simulink model "Harness_chart2"  (R2017b)
settings: Solver=VariableStepAuto  StartTime=0.0  StopTime=2  RelTol=1e-3
undefined symbols (not defined in the file): sigbuilder_block
settings Model: Creator=Kris  LastModifiedBy=Kris

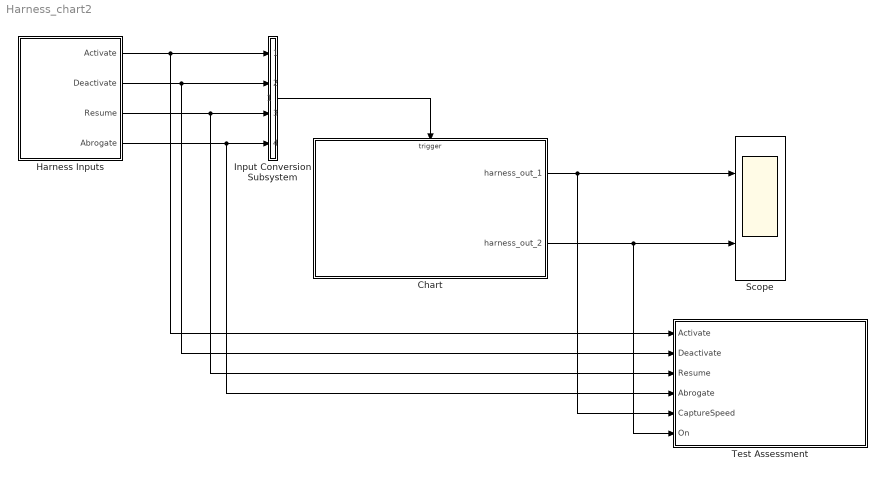
== system Harness_chart2 ==
  Chart : Subsystem  Tag=__SL_testing_harness_stub_
  Harness Inputs : Subsystem  Tag=STV Subsys  LoadFcn=sigbuilder_block('load');  StartFcn=sigbuilder_block('start');  StopFcn=sigbuilder_block('stop');  ClipboardFcn=sigbuilder_block('clipboard');  mask(Sigbuilder block){tuvar=[0:10]}
      mask init:
      | if ~strcmp(get_param(bdroot(gcb),'SimulationStatus'),'stopped'),tuvar = sigbuilder_block('maskInit'); end
      settings: CopyFcn=sigbuilder_block('copy');  DeleteFcn=sigbuilder_block('delete');  ModelCloseFcn=sigbuilder_block('modelClose');  PreSaveFcn=sigbuilder_block('preSave');  PauseFcn=sigbuilder_block('pause');  ContinueFcn=sigbuilder_block('continue');  NameChangeFcn=sigbuilder_block('namechange');  OpenFcn=sigbuilder_block('open',[50.25 50.25 717.75 399.75 ]);  CloseFcn=sigbuilder_block('close');
      mask Display: plot(0, 0, 100, 100,[2, 2, 32, 32, 2], [68, 8, 8, 68, 68],[32, 2], [38, 38], [32, 19, 2],[53, 60, 44], [32, 17, 17, 2],[16, 16, 31, 31]);txt = getActiveGroup(gcbh);text(2, 100, txt,'verticalAlignment', 'top');
  Input Conversion Subsystem : Subsystem  Tag=__SLT_ICS__  Description=|
      | Signal spec.
      | and routing
      settings: AttributesFormatString=%<Description>
  Scope : Scope  NumInputPorts=2
  Test Assessment : Test Sequence  TreatAsAtomicUnit=on
  wires:
  Harness Inputs/1(Activate) -> Test Assessment/1(Activate), Input Conversion Subsystem/1(Inport_1)
  Harness Inputs/2(Deactivate) -> Test Assessment/2(Deactivate), Input Conversion Subsystem/2(Inport_2)
  Harness Inputs/3(Resume) -> Test Assessment/3(Resume), Input Conversion Subsystem/3(Inport_3)
  Chart/2(harness_out_2) -> Test Assessment/6(On), Scope/2
  Input Conversion Subsystem/1(Outport_1) -> Chart/Trigger
  Chart/1(harness_out_1) -> Test Assessment/5(CaptureSpeed), Scope/1
  Harness Inputs/4(Abrogate) -> Test Assessment/4(Abrogate), Input Conversion Subsystem/4(Inport_4)

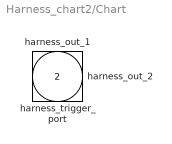
== system Harness_chart2/Chart ==
  harness_trigger_port : TriggerPort  VariantControl=(inherit)
  harness_out_1 : Outport
  harness_out_2 : Outport  Port=2

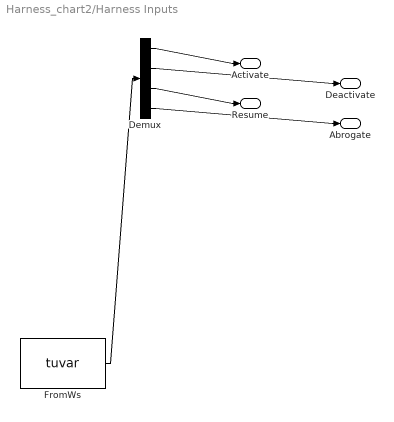
== system Harness_chart2/Harness Inputs ==
  Demux : Demux  Tag=STV Demux
  FromWs : FromWorkspace  Tag=STV FromWs  VariableName=tuvar  SampleTime=0
      SigBuilderData=|
      | dataSet.timeRange = [0 2]
      | dataSet.name = 'Group 1'
      | sbobj.Name = 'Signal Builder'
      | sbobj.Groups.Name = 'Group 1'
      | sbobj.Groups.Signals(1).Name = 'Activate'
      | sbobj.Groups.Signals(1).XData = [0 0.1 0.1 0.4 0.4 0.502 0.502 1 1 1.205 1.205 2]
      | sbobj.Groups.Signals(1).YData = [1 1 0 0 1 1 0 0 1 1 0 0]
      | sbobj.Groups.Signals(2).Name = 'Deactivate'
      | sbobj.Groups.Signals(2).XData = [0 0.1 0.1 0.2 0.2 0.606 0.698 1.615 1.615 1.755 1.755 2]
      | sbobj.Groups.Signals(2).YData = [0 0 1 1 0 0 0 0 1 1 0 0]
      | sbobj.Groups.Signals(3).Name = 'Resume'
      | sbobj.Groups.Signals(3).XData = [0 0.774 0.774 0.858 0.858 2]
      | sbobj.Groups.Signals(3).YData = [0 0 1 1 0 0]
      | sbobj.Groups.Signals(4).Name = 'Abrogate'
      | sbobj.Groups.Signals(4).XData = [0 0.598 0.598 0.696 0.696 1.205 1.205 1.405 1.405 2]
      | sbobj.Groups.Signals(4).YData = [0 0 1 1 0 0 1 1 0 0]
      | sbobj.Groups.TimeRange = [0 2]
  Activate : Outport  Tag=STV Outport
  Deactivate : Outport  Tag=STV Outport  Port=2
  Resume : Outport  Tag=STV Outport  Port=3
  Abrogate : Outport  Tag=STV Outport  Port=4
  wires:
  FromWs/1 -> Demux/1
  Demux/1 -> Activate/1
  Demux/2 -> Deactivate/1
  Demux/3 -> Resume/1
  Demux/4 -> Abrogate/1

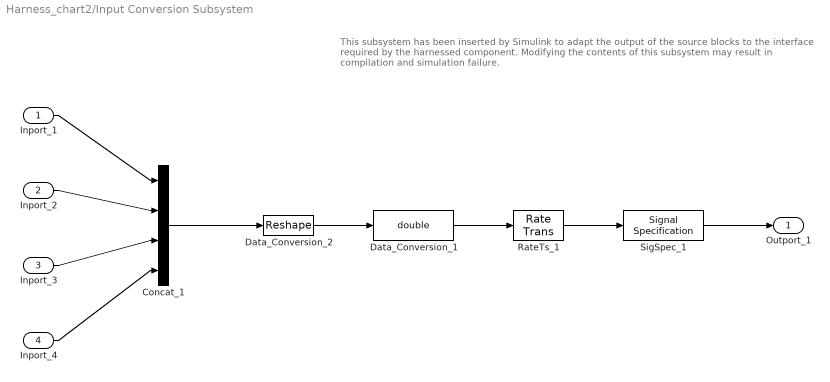
== system Harness_chart2/Input Conversion Subsystem ==
  note: This subsystem has been inserted by Simulink to adapt the output of the source blocks to the interface required by the harnessed component.
      |  Modifying the contents of this subsystem may result in compilation and simulation failure.
  Inport_1 : Inport
  Inport_2 : Inport  Port=2
  Inport_3 : Inport  Port=3
  Inport_4 : Inport  Port=4
  Concat_1 : Concatenate  NumInputs=4
  Data_Conversion_1 : DataTypeConversion  OutDataTypeStr=double  SaturateOnIntegerOverflow=on  RndMeth=Zero
  Data_Conversion_2 : Reshape  OutputDimensionality=Customize  OutputDimensions=[4]
  RateTs_1 : RateTransition  OutPortSampleTime=[-1, 0]
  SigSpec_1 : SignalSpecification  OutDataTypeStr=double  Dimensions=[4]  SampleTime=[-1, 0]
  Outport_1 : Outport
  wires:
  SigSpec_1/1 -> Outport_1/1
  RateTs_1/1 -> SigSpec_1/1
  Data_Conversion_1/1 -> RateTs_1/1
  Data_Conversion_2/1 -> Data_Conversion_1/1
  Concat_1/1 -> Data_Conversion_2/1
  Inport_1/1 -> Concat_1/1
  Inport_2/1 -> Concat_1/2
  Inport_3/1 -> Concat_1/3
  Inport_4/1 -> Concat_1/4

== stateflow chart Harness_chart2/Test Assessment ==
  settings: stateMachineType=SIMPLIFIED_MACHINE
  state Initialize_state_off
    verify(~On)
    verify(~CaptureSpeed)
    state step_1_1
    state step_1_2
    (default) -> (junction 22)
    Initialize_state_off -> (junction 22) [order 1]
    (junction 22) -> (junction 23) [order 1] : [t < 5]
    (junction 23) -> step_1_1 [order 1] : [~in(step_1_1)]
    (junction 23) -> (junction 26) [order 2]
    (junction 31) -> (junction 32)
    (junction 32) -> step_1_2 [order 1] : [~in(step_1_2)]
    (junction 32) -> (junction 35) [order 2]
    (junction 22) -> (junction 31) [order 2]
  state On
    verify(On>0)
    verify(CaptureSpeed>0)
  state Suspended
    verify(~On)
    verify(CaptureSpeed>0)
  (default) -> Initialize_state_off
  (junction 58) -> Initialize_state_off
  (junction 65) -> (junction 58)
  Initialize_state_off -> On [order 1] : [hasChangedTo(Activate,1)
      | ]
  On -> Initialize_state_off [order 1] : [hasChangedTo(Deactivate,1)
      | ]
  On -> Suspended [order 2] : [hasChangedTo(Abrogate,1)
      | ]
  Suspended -> On [order 2] : [hasChangedTo(Resume,1)
      | ]
  Suspended -> (junction 65) [order 1] : [hasChangedTo(Deactivate,1)
      | ]
  data: Activate input; Deactivate input; Resume input; Abrogate input; CaptureSpeed input; On input
